simulink model "baitn2"  (R2015a)
settings: Solver=ode45  StartTime=0.0  StopTime=20  RelTol=1e-3
libraries: simulink x1
settings Model: Creator=nguye  LastModifiedBy=nguye

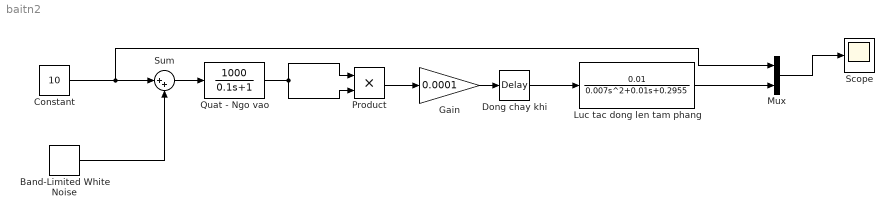
== system baitn2 ==
  Band-Limited White Noise : simulink/Sources/Band-Limited White Noise  Cov=[0.001]  Ts=0.1  seed=[23341]
  Constant : Constant  Value=10
  Dong chay khi : TransportDelay  DelayTime=0.1
  Gain : Gain  Gain=0.0001
  Luc tac dong len tam phang : TransferFcn  Numerator=[0.01]  Denominator=[0.007 0.01 0.2955]
  Mux : Mux  Inputs=2
  Product : Product
  Quat - Ngo vao : TransferFcn  Numerator=[1000]  Denominator=[0.1 1]
  Scope : Scope
  Sum : Sum  Inputs=|++
  wires:
  Sum/1 -> Quat - Ngo vao/1
  Product/1 -> Gain/1
  Gain/1 -> Dong chay khi/1
  Dong chay khi/1 -> Luc tac dong len tam phang/1
  Band-Limited White Noise/1 -> Sum/2
  Quat - Ngo vao/1 -> Product/2, Product/1
  Luc tac dong len tam phang/1 -> Mux/2
  Constant/1 -> Mux/1, Sum/1
  Mux/1 -> Scope/1
